simulink model "dyn_model"  (R2023b)
settings: Solver=VariableStepAuto  StartTime=0.0  StopTime=100  RelTol=1e-3
values from neighbouring files (symbols this model uses):
  A = double(A)    [consistent.m]    (also in dyn_model_mark.m)
  B = double(B)    [consistent.m]    (also in dyn_model_mark.m)
  C = [1 0 0 0 ... (first row only)    [consistent.m]    (also in dyn_model_mark.m)
  D = [0 ... (first row only)    [consistent.m]    (also in dyn_model_mark.m)
  den_phi = cell2mat(G_t2p.Denominator)    [consistent.m]    (also in dyn_model_mark.m)
  den_theta = cell2mat(G_ol.Denominator(1,1))    [consistent.m]    (also in dyn_model_mark.m)
  g0 = 9.81    [consistent.m]    (also in dyn_model_mark.m)
  Ip = (mp*Lp^2)/12    (= 3.3282e-05)    [consistent.m]    (also in dyn_model_mark.m = 8.3205e-06)
  Ir = (mr*Lr^2)/12    (= 5.71979166667e-05)    [consistent.m]    (also in dyn_model_mark.m = 1.42994791667e-05)
  J = 4e-6    (= 4e-06)    [consistent.m]    (also in dyn_model_mark.m)
  k = 42e-3    (= 0.042)    [consistent.m]    (also in dyn_model_mark.m)
  La = 1.16e-3    (= 0.00116)    [consistent.m]    (also in dyn_model_mark.m)
  Lp = 0.129    [consistent.m]    (also in dyn_model_mark.m = 0.0645)
  Lr = 0.085    [consistent.m]    (also in dyn_model_mark.m)
  mp = 0.024    [consistent.m]    (also in dyn_model_mark.m)
  mr = 0.095    [consistent.m]    (also in dyn_model_mark.m)
  num_phi = cell2mat(G_t2p.Numerator)    [consistent.m]    (also in dyn_model_mark.m)
  num_theta = cell2mat(G_ol.Numerator(1,1))    [consistent.m]    (also in dyn_model_mark.m)
  param = [mr mp Lr Lp Ir Ip g0]'    [consistent.m]    (also in dyn_model_mark.m)
  Ra = 8.4    [consistent.m]    (also in dyn_model_mark.m)
  Va_bar = double(sol)    [consistent.m]    (also in dyn_model_mark.m)
  x1_bar = 0    [consistent.m]    (also in dyn_model_mark.m)
  x3_bar = 0    [consistent.m]    (also in dyn_model_mark.m = 3.14159265359)
undefined symbols (not defined in the file or in its folder): rot_pend
libraries: simulink_extras x2, simulink x2
settings Model: Creator=Mark  LastModifiedBy=Mark
settings OptimizationCC: BlockReduction=off  DefaultParameterBehavior=Inlined  BufferReuse=off

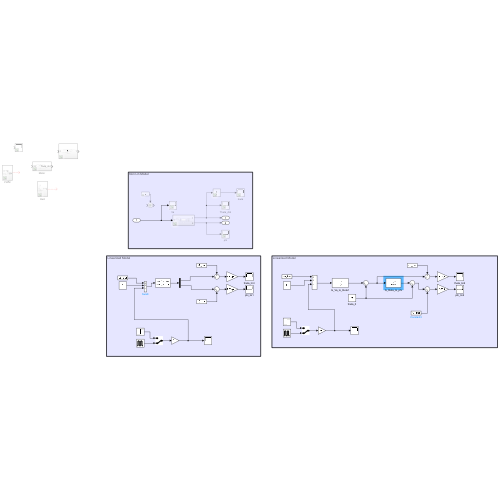
[thumbnail: Simulink's stored preview of the top-level diagram]
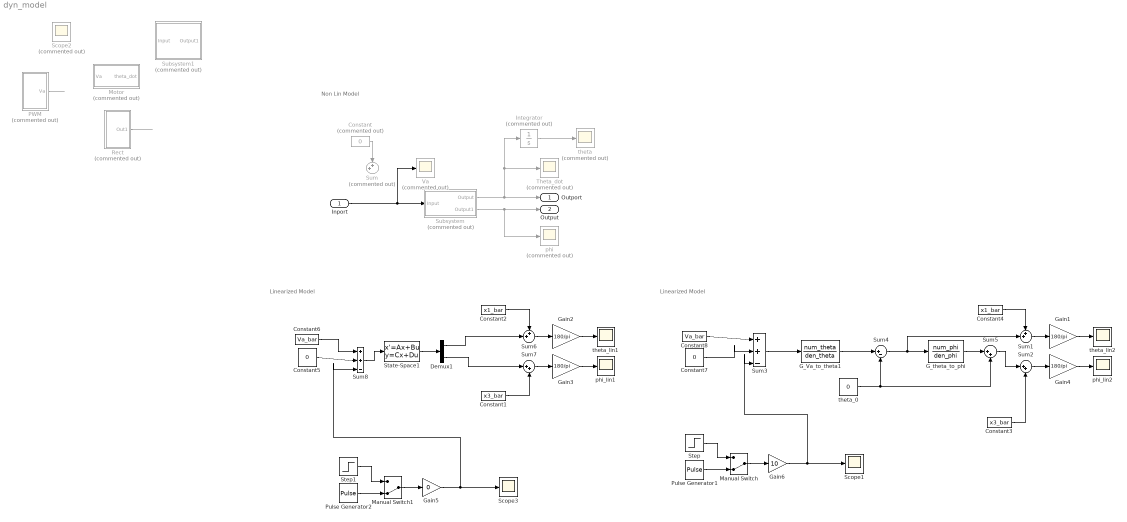
== system dyn_model ==
  note: Non Lin Model
  note: Linearized Model
  note: Linearized Model
  Inport : Inport
  Constant : Constant  Commented=on  Value=0
  Constant1 : Constant  Value=x3_bar
  Constant2 : Constant  Value=x1_bar
  Constant3 : Constant  Value=x3_bar
  Constant4 : Constant  Value=x1_bar
  Constant5 : Constant  Value=0
  Constant6 : Constant  Value=Va_bar
  Constant7 : Constant  Value=0
  Constant8 : Constant  Value=Va_bar
  Demux1 : Demux  Outputs=2
  G_Va_to_theta1 : TransferFcn  Numerator=num_theta  Denominator=den_theta
  G_theta_to_phi : TransferFcn  Numerator=num_phi  Denominator=den_phi
  Gain{1..4} (4 alike) : Gain  Gain=180/pi
  Gain5 : Gain  Gain=0
  Gain6 : Gain  Gain=10
  Integrator : Integrator  Commented=on
  Manual Switch : ManualSwitch  CurrentSetting=0
  Manual Switch1 : ManualSwitch  CurrentSetting=0
  Motor : Subsystem  Commented=on
  PWM : Subsystem  Commented=on
  Pulse Generator1 : DiscretePulseGenerator  PulseType=Time based  Period=10000  PulseWidth=0.001  PhaseDelay=1
  Pulse Generator2 : DiscretePulseGenerator  PulseType=Time based  Period=10000  PulseWidth=0.001  PhaseDelay=1
  Rect : Subsystem  Commented=on
  Scope1 : Scope
  Scope2 : Scope  Commented=on
  Scope3 : Scope
  State-Space1 : StateSpace  A=A  B=B  C=C  D=D  InitialCondition=[0 0 pi/2 0]  ParameterTunability=Optimized
  Step : Step  Time=20  SampleTime=0
  Step1 : Step  Time=20  SampleTime=0
  Subsystem : Subsystem  Commented=on
  Subsystem1 : Subsystem  Commented=on
  Sum : Sum  Commented=on  Inputs=++|
  Sum1 : Sum  Inputs=++|
  Sum2 : Sum  Inputs=|++
  Sum3 : Sum  Inputs=++-|
  Sum4 : Sum  Inputs=|+-
  Sum5 : Sum  Inputs=|++
  Sum6 : Sum  Inputs=++|
  Sum7 : Sum  Inputs=|++
  Sum8 : Sum  Inputs=++-|
  Theta_dot : Scope  Commented=on
  Va : Scope  Commented=on
  phi : Scope  Commented=on
  phi_lin1 : Scope
  phi_lin2 : Scope
  theta : Scope  Commented=on
  theta_0 : Constant  Value=0
  theta_lin1 : Scope
  theta_lin2 : Scope
  Outport : Outport
  Output : Outport  Port=2
  wires:
  PWM/1(Va) -> ?
  Subsystem/1(Output) -> Outport/1, Integrator/1, Theta_dot/1
  Subsystem/2(Output1) -> phi/1, Output/1
  Inport/1 -> Va/1, Subsystem/1(Input)
  Integrator/1 -> theta/1
  Rect/1(Out1) -> ?
  Constant/1 -> Sum/1
  Constant6/1 -> Sum8/1
  Sum6/1 -> Gain2/1
  Constant1/1 -> Sum7/2
  Constant2/1 -> Sum6/1
  Gain3/1 -> phi_lin1/1
  Demux1/2 -> Sum7/1
  Sum7/1 -> Gain3/1
  Constant5/1 -> Sum8/2
  State-Space1/1 -> Demux1/1
  Demux1/1 -> Sum6/2
  Sum8/1 -> State-Space1/1
  Gain2/1 -> theta_lin1/1
  Gain1/1 -> theta_lin2/1
  Sum1/1 -> Gain1/1
  Sum4/1 -> Sum1/2, G_theta_to_phi/1
  Sum5/1 -> Sum2/1
  Constant3/1 -> Sum2/2
  Constant7/1 -> Sum3/2
  Constant8/1 -> Sum3/1
  Sum2/1 -> Gain4/1
  Constant4/1 -> Sum1/1
  Gain4/1 -> phi_lin2/1
  Sum3/1 -> G_Va_to_theta1/1
  Manual Switch/1 -> Gain6/1
  Pulse Generator1/1 -> Manual Switch/2
  Gain6/1 -> Sum3/3, Scope1/1
  Step/1 -> Manual Switch/1
  Gain5/1 -> Sum8/3, Scope3/1
  Manual Switch1/1 -> Gain5/1
  Pulse Generator2/1 -> Manual Switch1/2
  Step1/1 -> Manual Switch1/1
  G_Va_to_theta1/1 -> Sum4/1
  theta_0/1 -> Sum5/2, Sum4/2
  G_theta_to_phi/1 -> Sum5/1

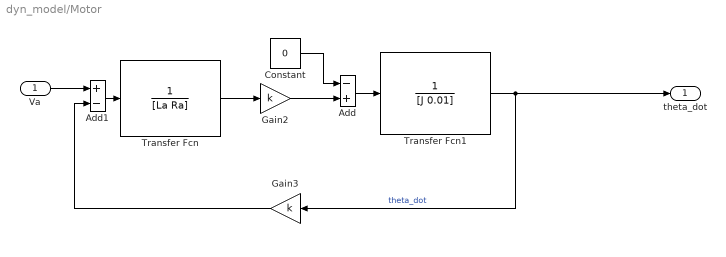
== system dyn_model/Motor ==
  Va : Inport
  Add : Sum  Inputs=-+
  Add1 : Sum  Inputs=+-
  Constant : Constant  Value=0
  Gain2 : Gain  Gain=k
  Gain3 : Gain  Gain=k
  Transfer Fcn : TransferFcn  Denominator=[La Ra]
  Transfer Fcn1 : TransferFcn  Denominator=[J 0.01]
  theta_dot : Outport
  wires:
  Gain3/1 -> Add1/2
  Transfer Fcn1/1 -> theta_dot/1, Gain3/1  "theta_dot"
  Add1/1 -> Transfer Fcn/1
  Va/1 -> Add1/1
  Constant/1 -> Add/1
  Gain2/1 -> Add/2
  Add/1 -> Transfer Fcn1/1
  Transfer Fcn/1 -> Gain2/1

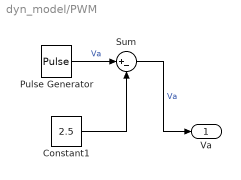
== system dyn_model/PWM ==
  Constant1 : Constant  Value=2.5
  Pulse Generator : DiscretePulseGenerator  PulseType=Time based  Amplitude=5  Period=10  PulseWidth=50
  Sum : Sum  Inputs=|+-
  Va : Outport
  wires:
  Pulse Generator/1 -> Sum/1  "Va"
  Constant1/1 -> Sum/2
  Sum/1 -> Va/1  "Va"

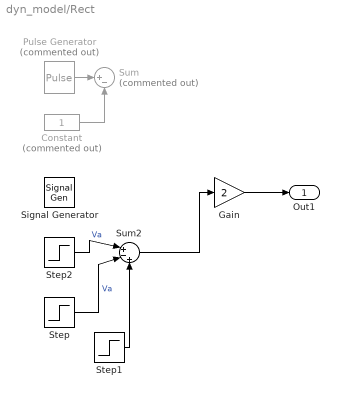
== system dyn_model/Rect ==
  Constant : Constant  Commented=on
  Gain : Gain  Gain=2
  Pulse Generator : DiscretePulseGenerator  Commented=on  PulseType=Time based  Amplitude=2  Period=1  PulseWidth=50  PhaseDelay=1
  Signal Generator : SignalGenerator  WaveForm=square  Amplitude=1.8  Frequency=0.5  Units=rad/sec
  Step : Step  Time=1.5  After=2  SampleTime=0
  Step1 : Step  Time=2  SampleTime=0
  Step2 : Step  SampleTime=0
  Sum : Sum  Commented=on  Inputs=|+-
  Sum2 : Sum  Inputs=|+-+
  Out1 : Outport
  wires:
  Step2/1 -> Sum2/1  "Va"
  Step/1 -> Sum2/2  "Va"
  Sum2/1 -> Gain/1
  Gain/1 -> Out1/1
  Constant/1 -> Sum/2
  Step1/1 -> Sum2/3
  Pulse Generator/1 -> Sum/1

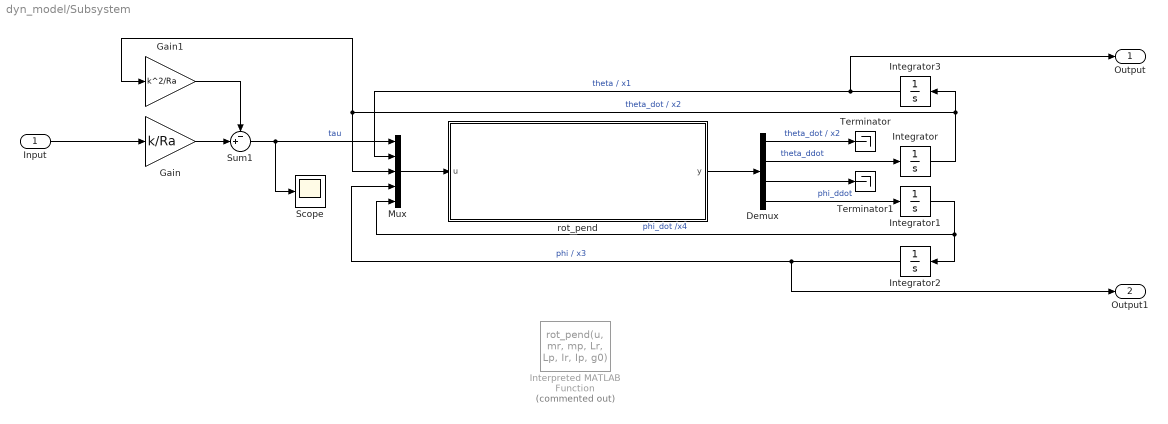
== system dyn_model/Subsystem ==
  Input : Inport
  Demux : Demux
  Gain : Gain  Gain=k/Ra
  Gain1 : Gain  Gain=k^2/Ra
  Integrator{,1..3} (4 alike) : Integrator
  Interpreted MATLAB Function : MATLABFcn  Commented=on  MATLABFcn=rot_pend(u, mr, mp, Lr, Lp, Ir, Ip, g0)  OutputDimensions=4  OutputSignalType=real
  Mux : Mux  Inputs=5
  Scope : Scope
  Sum1 : Sum  Inputs=-+|
  Terminator : Terminator
  Terminator1 : Terminator
  rot_pend : Subsystem
  Output : Outport
  Output1 : Outport  Port=2
  wires:
  Sum1/1 -> Scope/1, Mux/1  "tau"
  Integrator2/1 -> Output1/1, Mux/4  "phi / x3"
  Integrator/1 -> Integrator3/1, Mux/3, Gain1/1  "theta_dot / x2"
  Mux/1 -> rot_pend/1(u)
  rot_pend/1(y) -> Demux/1
  Gain/1 -> Sum1/2
  Integrator1/1 -> Mux/5, Integrator2/1  "phi_dot /x4"
  Gain1/1 -> Sum1/1
  Integrator3/1 -> Mux/2, Output/1  "theta / x1"
  Demux/4 -> Integrator1/1  "phi_ddot"
  Input/1 -> Gain/1
  Demux/2 -> Integrator/1  "theta_ddot"
  Demux/1 -> Terminator/1  "theta_dot / x2"
  Demux/3 -> Terminator1/1

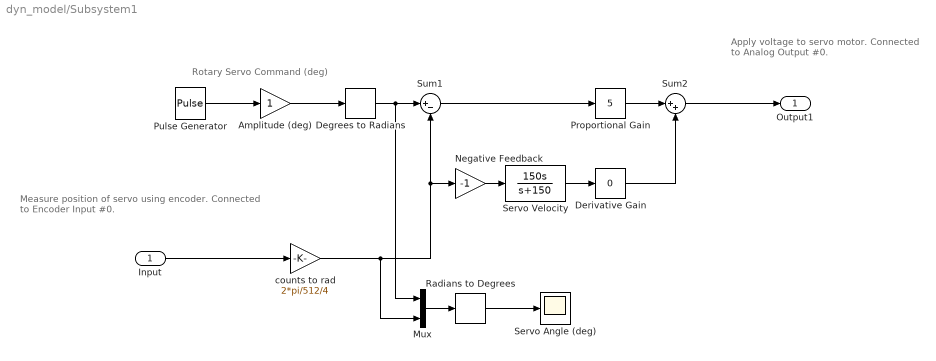
== system dyn_model/Subsystem1 ==
  note: Measure position of servo using encoder.
      | Connected to Encoder Input #0.
  note: Rotary Servo Command (deg)
  note: Apply voltage to servo motor.
      | Connected to Analog Output #0.
  Input : Inport
  Amplitude (deg) : Gain
  Degrees to Radians : simulink_extras/Transformations/Degrees to Radians
  Derivative Gain : simulink/Math Operations/Slider Gain  gain=0  low=0  high=0.5
  Mux : Mux  Inputs=2
  Negative Feedback : Gain  Gain=-1
  Proportional Gain : simulink/Math Operations/Slider Gain  gain=5  low=1  high=10
  Pulse Generator : DiscretePulseGenerator  PulseType=Time based  Amplitude=90  Period=10  PulseWidth=50
  Radians to Degrees : simulink_extras/Transformations/Radians to Degrees
  Servo Angle (deg) : Scope
  Servo Velocity : TransferFcn  Numerator=[150 0]  Denominator=[1 150]
  Sum1 : Sum  Inputs=|+-
  Sum2 : Sum  Inputs=|++
  counts to rad : Gain  Gain=2*pi/512/4
  Output1 : Outport
  wires:
  Negative Feedback/1 -> Servo Velocity/1
  Degrees to Radians/1 -> Sum1/1, Mux/1
  Amplitude (deg)/1 -> Degrees to Radians/1
  Derivative Gain/1 -> Sum2/2
  Servo Velocity/1 -> Derivative Gain/1
  Mux/1 -> Radians to Degrees/1
  Pulse Generator/1 -> Amplitude (deg)/1
  Sum1/1 -> Proportional Gain/1
  Radians to Degrees/1 -> Servo Angle (deg)/1
  counts to rad/1 -> Sum1/2, Negative Feedback/1, Mux/2
  Input/1 -> counts to rad/1
  Proportional Gain/1 -> Sum2/1
  Sum2/1 -> Output1/1

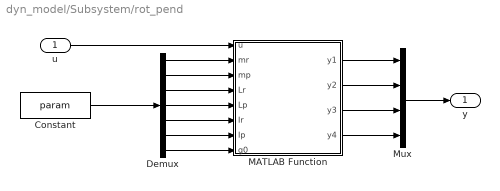
== system dyn_model/Subsystem/rot_pend ==
  u : Inport
  Constant : Constant  Value=param  VectorParams1D=off
  Demux : Demux  Outputs=7
  MATLAB Function : MATLAB Function  TreatAsAtomicUnit=on
  Mux : Mux
  y : Outport
  wires:
  Demux/3 -> MATLAB Function/4(Lr)
  Demux/5 -> MATLAB Function/6(Ir)
  Demux/4 -> MATLAB Function/5(Lp)
  Demux/7 -> MATLAB Function/8(g0)
  Demux/2 -> MATLAB Function/3(mp)
  Demux/6 -> MATLAB Function/7(Ip)
  Demux/1 -> MATLAB Function/2(mr)
  u/1 -> MATLAB Function/1(u)
  Constant/1 -> Demux/1
  MATLAB Function/1(y1) -> Mux/1
  MATLAB Function/2(y2) -> Mux/2
  MATLAB Function/3(y3) -> Mux/3
  MATLAB Function/4(y4) -> Mux/4
  Mux/1 -> y/1

== matlab function dyn_model/Subsystem/rot_pend/MATLAB Function ==
  data: u input; y1 output; mr input; mp input; Lr input; Lp input; Ir input; Ip input; g0 input; y2 output; y3 output; y4 output
function [y1,y2,y3,y4] = rot_pend(u, mr, mp, Lr, Lp, Ir, Ip, g0)
%UNTITLED Summary of this function goes here
%   Detailed explanation goes here
% u(1) = Va
x1 = u(2) ; % theta
x2 = u(3) ; % theta_dot
x3 = u(4) ; % phi
x4 = u(5) ; % phi_dot

a = mr*(Lr/2)^2 + mp*(Lr^2+(Lp*sin(x3))^2) + Ir ;
b = mp*Lr*Lp*cos(x3) ;
%c = b ;
d = mp*Lp^2+Ip ;

e = (-2*mp*Lp^2*sin(x3)*cos(x3)*x2*x4) + ( mp*Lr*Lp*sin(x3)*x2^2 ) + u(1) ;
f = ( mp*Lp^2*sin(x3)*cos(x3)*x2^2 ) + ( mp*g0*Lp*sin(x3) ) ;

B = [a b;
     b d] ;
ne = [e f]' ;
q_ddot = B\ne ;

y1 = x2 ;
y2 = q_ddot(1) ;
y3 = x4 ;
y4 = q_ddot(2) ;
